simulink model "untitled"  (R2017a)
settings: Solver=VariableStepAuto  StartTime=0.0  StopTime=10.0  RelTol=1e-3
undefined symbols (not defined in the file): a, r
libraries: simulink x1
settings Model: Creator=Anton  LastModifiedBy=Anton

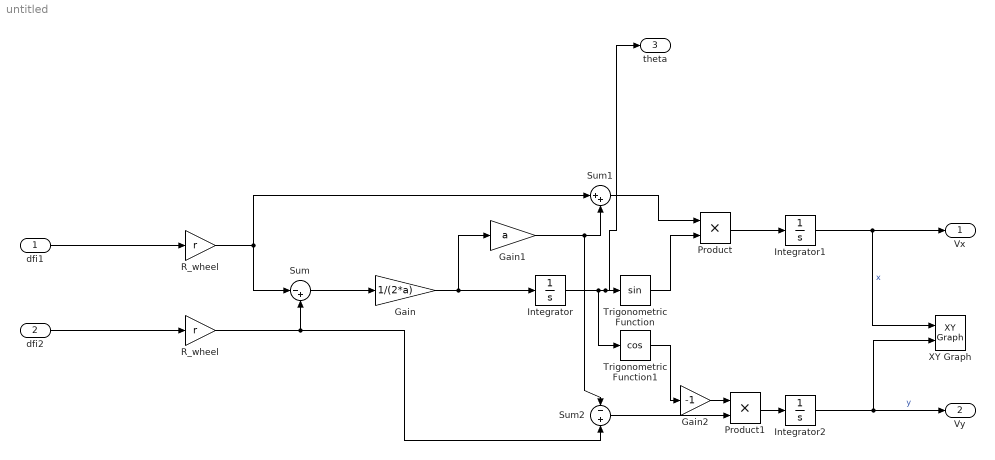
== system untitled ==
  dfi1 : Inport
  dfi2 : Inport  Port=2
  Gain : Gain  Gain=1/(2*a)
  Gain1 : Gain  Gain=a
  Gain2 : Gain  Gain=-1
  Integrator : Integrator
  Integrator1 : Integrator
  Integrator2 : Integrator
  Product : Product
  Product1 : Product
  R_wheel : Gain  Gain=r
  "R_wheel " : Gain  Gain=r
  Sum : Sum  Inputs=|-+
  Sum1 : Sum  Inputs=|++
  Sum2 : Sum  Inputs=-+
  Trigonometric Function : Trigonometry
  Trigonometric Function1 : Trigonometry  Operator=cos
  XY Graph : simulink/Sinks/XY Graph  xmin=-1  xmax=1  ymin=-1  ymax=1  st=-1
  Vx : Outport
  Vy : Outport  Port=2
  theta : Outport  Port=3
  wires:
  dfi1/1 -> R_wheel/1
  dfi2/1 -> "R_wheel "/1
  R_wheel/1 -> Sum/1, Sum1/1
  "R_wheel "/1 -> Sum2/2, Sum/2
  Sum/1 -> Gain/1
  Gain/1 -> Integrator/1, Gain1/1
  Gain1/1 -> Sum1/2, Sum2/1
  Integrator/1 -> theta/1, Trigonometric Function/1, Trigonometric Function1/1
  Sum1/1 -> Product/1
  Trigonometric Function/1 -> Product/2
  Trigonometric Function1/1 -> Gain2/1
  Sum2/1 -> Product1/2
  Product/1 -> Integrator1/1
  Product1/1 -> Integrator2/1
  Integrator1/1 -> XY Graph/1, Vx/1  "x"
  Integrator2/1 -> XY Graph/2, Vy/1  "y"
  Gain2/1 -> Product1/1
